simulink model "Lab3_zad2_old"  (R2018a)
settings: Solver=ode4  StartTime=0.0  StopTime=SimTime  FixedStep=0.01  RelTol=1e-3  EnableMultiTasking=on
values from neighbouring files (symbols this model uses):
  A = (1+r/m)^(m*n)    (= 1.12699211369)    [Script.m]
  AP = expm(A*Step)    [Script.m]
  B = 0    [Script.m]
  BP = double(vpaintegral(fun,t,[0 Step])) * B    [Script.m]
  C = 1    [Script.m]
  D = 0    [Script.m]
  IC = 10    [Script.m]
  Step = 1/m    (= 0.25)    [Script.m]
settings Model: Creator=falcon  LastModifiedBy=falcon
settings SolverCC: AutoInsertRateTranBlk=on
settings DataIOCC: LimitDataPoints=on  ReturnWorkspaceOutputs=on
settings SFSimCC: SimUseLocalCustomCode=on
settings RTWCC: RTWUseLocalCustomCode=on

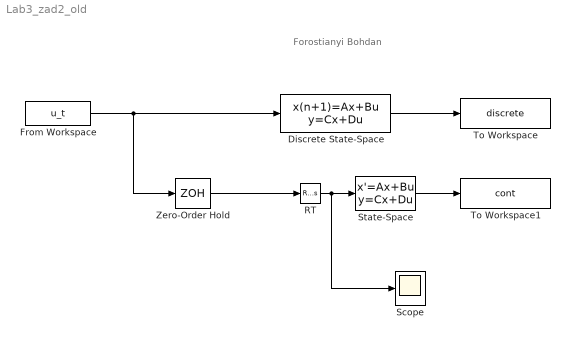
== system Lab3_zad2_old ==
  note: Forostianyi Bohdan
  Discrete State-Space : DiscreteStateSpace  A=AP  B=BP  C=C  D=D  InitialCondition=IC  SampleTime=-1
  From Workspace : FromWorkspace  VariableName=u_t  SampleTime=Step
  RT : RateTransition  OutPortSampleTime=0.01
  Scope : Scope
  State-Space : StateSpace  A=A  B=B  C=C  D=D  InitialCondition=IC
  To Workspace : ToWorkspace  VariableName=discrete  SaveFormat=Timeseries  SampleTime=-1
      settings: Save2DSignal=2-D array (concatenate along first dimension)
  To Workspace1 : ToWorkspace  VariableName=cont  SaveFormat=Timeseries  SampleTime=-1
  Zero-Order Hold : ZeroOrderHold  SampleTime=Step
  wires:
  From Workspace/1 -> Discrete State-Space/1, Zero-Order Hold/1
  Discrete State-Space/1 -> To Workspace/1
  Zero-Order Hold/1 -> RT/1
  State-Space/1 -> To Workspace1/1
  RT/1 -> Scope/1, State-Space/1
